simulink subsystem "ControladorBA"  (R2023b)
settings: Solver=VariableStepAuto  StartTime=0.0  StopTime=10.0  RelTol=1e-3
settings Model: Creator=USUARIO  LastModifiedBy=USUARIO

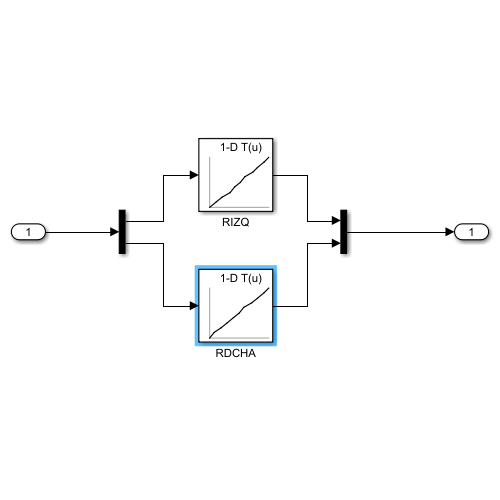
[thumbnail: Simulink's stored preview of the top-level diagram]
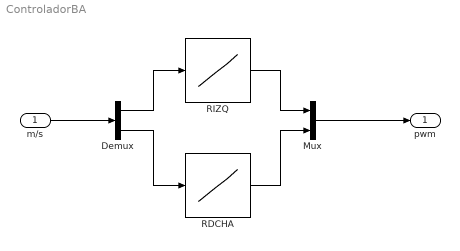
== system ControladorBA ==
  m/s : Inport
  Demux : Demux  Outputs=2
  Mux : Mux  Inputs=2
  RDCHA : Lookup_n-D  NumberOfTableDimensions=1  BreakpointsForDimension1=[-0.352425247430801 -0.290246039628983 -0.217681556940079 -0.145123019814491 -0.062193028628826 0 0.051828362047672 0.145119562745094 0.217674165964127 0.300605893135071 0.352433651685715]  Table=[-255 -200 -150 -100 -50 0 50 100 150 200 255]  InternalRulePriority=Speed  RndMeth=Simplest
  RIZQ : Lookup_n-D  NumberOfTableDimensions=1  BreakpointsForDimension1=[-0.362790256738663 -0.279880553483963 -0.217687517404556 -0.124386087059975 -0.062193028628826 0 0.051828384399414 0.145119190216064 0.196943387389183 0.279873877763748 0.331700176000595]  Table=[-255 -200 -150 -100 -50 0 50 100 150 200 255]  InternalRulePriority=Speed  RndMeth=Simplest
  pwm : Outport
  wires:
  m/s/1 -> Demux/1
  Mux/1 -> pwm/1
  Demux/2 -> RDCHA/1
  RDCHA/1 -> Mux/2
  Demux/1 -> RIZQ/1
  RIZQ/1 -> Mux/1
